simulink model "Delta_Inshallah_15RAMADAN"  (R2023b)
settings: Solver=VariableStepAuto  StartTime=1  StopTime=9  RelTol=1e-3
model workspace: external: MATLAB File D:\College\Senior 2\GP\Delta\Design\INSHALLAAHHHHH\SSCPE\25Mar\Ignorant_DataFile.m (data not in the file)
values from neighbouring files (symbols this model uses):
  X = [0 -180 -180 -180 180 180 180 180 0]    [Simulaiton_Main.m]    (also in csp_XYZ.m; csp_XYZ_X.m = [-180 -180]; csp_XYZ_circular_motion.m = center(1) + radius * cos(theta); csp_angles.m)
  Y = zeros(1,numel(X_3ars))    [CSPPPPPPPPPPPPpp.m]    (also in Simulaiton_Main.m = zeros(1,9); csp_XYZ.m = zeros(1,9); csp_XYZ_X.m = [0 0]; csp_XYZ_circular_motion.m = center(2) + radius * sin(theta))
  Z = -400*ones(1,numel(X_3ars))    [CSPPPPPPPPPPPPpp.m]    (also in Simulaiton_Main.m = [-300 -300 -400 -300 -300 -300 -400 -300 -300]; csp_XYZ.m = [-300 -300 -400 -300 -300 -300 -400 -300 -300]; csp_XYZ_X.m = [-300 -500]; csp_XYZ_circular_motion.m = center(3) * ones(size(X)))
undefined symbols (not defined in the file or in its folder): smiData
libraries: sm_lib x390, nesl_utility x4
(part 9 of 9)

== matlab function Delta_Inshallah_15RAMADAN/Trajectory Planning 1/Trajectory block1 ==
  data: q output; qdot output; q2dot output; t input; qt0 input; qtf input; delta_t input
function [q,qdot,q2dot] = trajectory_planning(t,qt0,qtf,delta_t)
t0=0;
tf = t0 + delta_t;
%qt0=-2*pi/6;
%qtf=pi/6;


qdott0=0;
qdottf=0;

A=[1 t0  t0^2 t0^3;
    0 1 2*t0 3*t0^2;
    1 tf tf^2 tf^3;
    0 1 2*tf 3*tf^2];

RHS=[qt0;qdott0;qtf;qdottf];

coeffs=inv(A)*RHS;

%t=linspace(t0,tf,100);
q=coeffs(4)*t.^3+coeffs(3)*t.^2+coeffs(2)*t+coeffs(1);
qdot=3*coeffs(4)*t.^2+2*coeffs(3)*t+coeffs(2);
q2dot=6*coeffs(4)*t+2*coeffs(3);

== matlab function Delta_Inshallah_15RAMADAN/Trajectory Planning 1/Trajectory block2 ==
  data: q output; qdot output; q2dot output; t input; qt0 input; qtf input; delta_t input
function [q,qdot,q2dot] = trajectory_planning(t,qt0,qtf,delta_t)
t0=0;
tf = t0 + delta_t;
%qt0=-2*pi/6;
%qtf=pi/6;


qdott0=0;
qdottf=0;

A=[1 t0  t0^2 t0^3;0 1 2*t0 3*t0^2;1 tf tf^2 tf^3;0 1 2*tf 3*tf^2];
RHS=[qt0;qdott0;qtf;qdottf];

coeffs=inv(A)*RHS;

%t=linspace(t0,tf,100);
q=coeffs(4)*t.^3+coeffs(3)*t.^2+coeffs(2)*t+coeffs(1);
qdot=3*coeffs(4)*t.^2+2*coeffs(3)*t+coeffs(2);
q2dot=6*coeffs(4)*t+2*coeffs(3);
